simulink model "Wyparka3"  (R2018a)
settings: Solver=ode45  StartTime=0.0  StopTime=1600  FixedStep=0.1  RelTol=1e-6  EnableMultiTasking=on
libraries: simulink x7
settings Model: Creator=Maciek  LastModifiedBy=klukomski
settings DataIOCC: SaveFormat=Array  SignalLoggingSaveFormat=ModelDataLogs
settings OptimizationCC: ExpressionDepthLimit=2147483647  LifeSpan=inf
settings DebuggingCC: UnderspecifiedInitializationDetection=Classic  MergeDetectMultiDrivingBlocksExec=none  SolverPrmCheckMsg=warning  FcnCallInpInsideContextMsg=warning  StateNameClashWarn=warning  SFUnexpectedBacktrackingDiag=warning  SFNoUnconditionalDefaultTransitionDiag=warning  SFExecutionAtInitializationDiag=none
settings HardwareCC: ProdBitPerPointer=32  ProdBitPerSizeT=32  ProdBitPerPtrDiffT=32  ProdLargestAtomicFloat=None  ProdIntDivRoundTo=Undefined  ProdEndianess=Unspecified  ProdWordSize=32  ProdHWDeviceType=32-bit Generic
settings ModelReferenceCC: PropagateSignalLabelsOutOfModel=off
settings CodeAppCC: StateflowObjectComments=on
settings GRTTargetCC: TargetLangStandard=C89/C90 (ANSI)  GeneratePreprocessorConditionals=Disable all  CombineOutputUpdateFcns=off  GRTInterface=on
settings ConfigComp: CovMetricSettings=dw  CovHtmlReporting=on  CovSaveCumulativeToWorkspaceVar=on  CovSaveSingleToWorkspaceVar=on  CovExternalEMLEnable=off

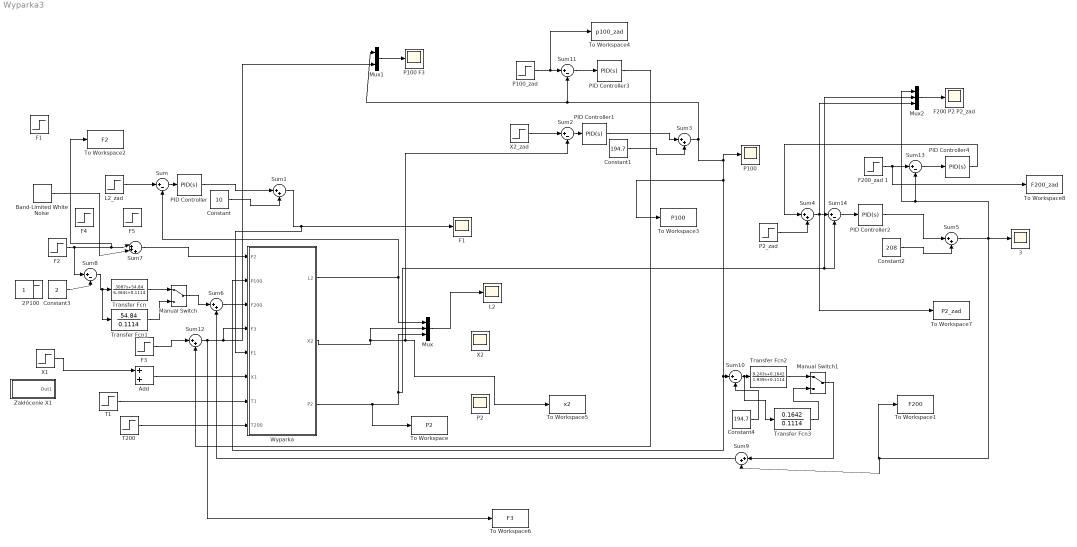
== system Wyparka3 ==
  "3 " : Scope
  Add : Sum
  Band-Limited White Noise : simulink/Sources/Band-Limited White Noise  Cov=[0.005]  Ts=2  seed=[23341]
  Constant : Constant  Value=10
  Constant1 : Constant  Value=194.7
  Constant2 : Constant  Value=208
  Constant3 : Constant  Value=2
  Constant4 : Constant  Value=194.7
  F1 : Step  Time=0  Before=10  After=9.9  SampleTime=0
  "F1 " : Scope
  F2 : Step  Time=200  Before=2  After=2  SampleTime=0
  F200 P2 P2_zad : Scope
  F200_zad 1 : Step  Time=700  Before=208  After=170  SampleTime=0
  F3 : Step  Time=0  Before=50  After=50  SampleTime=0
  F4 : Step  Time=300  After=-0.2  SampleTime=0
  F5 : Step  Time=2000  After=0.2  SampleTime=0
  L2 : Scope
  L2_zad : Step  Time=0  Before=1  SampleTime=0
  Manual Switch : ManualSwitch
  Manual Switch1 : ManualSwitch
  Mux : Mux  Inputs=3
  Mux1 : Mux  Inputs=2
  Mux2 : Mux  Inputs=3
  P100 : Step  Time=0  Before=194.7  After=194.7  SampleTime=0
  "P100 " : Scope
  P100 F3 : Scope
  "P100_zad " : Step  Time=100  Before=194.7  After=160  SampleTime=0
  P2 : Scope
  P2_zad : Step  Time=0  Before=50.5  After=50.5  SampleTime=0
  PID Controller : simulink/Continuous/PID Controller  Controller=PID  TimeDomain=Continuous-time  SampleTime=-1  IntegratorMethod=Forward Euler  FilterMethod=Forward Euler  Form=Parallel  UseFilter=on  ControllerParametersSource=internal  P=3.5228451242971  I=0.312459565800729  D=9.32811880876694  N=2.98089327538522  InitialConditionSource=internal  InitialConditionForIntegrator=0  InitialConditionForFilter=0  ExternalReset=none  LimitOutput=on  UpperSaturationLimit=10  LowerSaturationLimit=-10  LinearizeAsGain=on  AntiWindupMode=none  Kb=1  TrackingMode=off  Kt=1  PParamMin=[]  PParamMax=[]  IParamMin=[]  IParamMax=[]  DParamMin=[]  DParamMax=[]  NParamMin=[]  NParamMax=[]  KbParamMin=[]  KbParamMax=[]  KtParamMin=[]  KtParamMax=[]  POutMin=[]  POutMax=[]  IOutMin=[]  IOutMax=[]  DOutMin=[]  DOutMax=[]  NOutMin=[]  NOutMax=[]  KbOutMin=[]  KbOutMax=[]  KtOutMin=[]  KtOutMax=[]  IntegratorOutMin=[]  IntegratorOutMax=[]  FilterOutMin=[]  FilterOutMax=[]  SumOutMin=[]  SumOutMax=[]  SumI1OutMin=[]  SumI1OutMax=[]  SumI2OutMin=[]  SumI2OutMax=[]  SumI3OutMin=[]  SumI3OutMax=[]  SumDOutMin=[]  SumDOutMax=[]  SaturationOutMin=[]  SaturationOutMax=[]  IntegratorContinuousStateAttributes=''  IntegratorStateMustResolveToSignalObject=off  IntegratorRTWStateStorageClass=Auto  FilterContinuousStateAttributes=''  FilterStateMustResolveToSignalObject=off  FilterRTWStateStorageClass=Auto  DifferentiatorICPrevScaledInput=0  DifferentiatorOutMin=[]  DifferentiatorOutMax=[]  FilterDiffOutCoefMin=[]  FilterDiffOutCoefMax=[]  SumDenOutMin=[]  SumDenOutMax=[]  SumNumOutMin=[]  SumNumOutMax=[]  ReciprocalOutMin=[]  ReciprocalOutMax=[]  DivideOutMin=[]  DivideOutMax=[]  TunerSelectOption=Transfer Function Based (PID Tuner App)
  PID Controller1 : simulink/Continuous/PID Controller  Controller=PID  TimeDomain=Continuous-time  SampleTime=-1  IntegratorMethod=Forward Euler  FilterMethod=Forward Euler  Form=Parallel  UseFilter=on  ControllerParametersSource=internal  P=362.743618010896  I=63.281674643677  D=154.013703134731  N=5.51481835403711  InitialConditionSource=internal  InitialConditionForIntegrator=0  InitialConditionForFilter=0  ExternalReset=none  LimitOutput=on  UpperSaturationLimit=400-194.7  LowerSaturationLimit=-194.7  LinearizeAsGain=on  AntiWindupMode=none  Kb=1  TrackingMode=off  Kt=1  PParamMin=[]  PParamMax=[]  IParamMin=[]  IParamMax=[]  DParamMin=[]  DParamMax=[]  NParamMin=[]  NParamMax=[]  KbParamMin=[]  KbParamMax=[]  KtParamMin=[]  KtParamMax=[]  POutMin=[]  POutMax=[]  IOutMin=[]  IOutMax=[]  DOutMin=[]  DOutMax=[]  NOutMin=[]  NOutMax=[]  KbOutMin=[]  KbOutMax=[]  KtOutMin=[]  KtOutMax=[]  IntegratorOutMin=[]  IntegratorOutMax=[]  FilterOutMin=[]  FilterOutMax=[]  SumOutMin=[]  SumOutMax=[]  SumI1OutMin=[]  SumI1OutMax=[]  SumI2OutMin=[]  SumI2OutMax=[]  SumI3OutMin=[]  SumI3OutMax=[]  SumDOutMin=[]  SumDOutMax=[]  SaturationOutMin=[]  SaturationOutMax=[]  IntegratorContinuousStateAttributes=''  IntegratorStateMustResolveToSignalObject=off  IntegratorRTWStateStorageClass=Auto  FilterContinuousStateAttributes=''  FilterStateMustResolveToSignalObject=off  FilterRTWStateStorageClass=Auto  DifferentiatorICPrevScaledInput=0  DifferentiatorOutMin=[]  DifferentiatorOutMax=[]  FilterDiffOutCoefMin=[]  FilterDiffOutCoefMax=[]  SumDenOutMin=[]  SumDenOutMax=[]  SumNumOutMin=[]  SumNumOutMax=[]  ReciprocalOutMin=[]  ReciprocalOutMax=[]  DivideOutMin=[]  DivideOutMax=[]  TunerSelectOption=Transfer Function Based (PID Tuner App)
  PID Controller2 : simulink/Continuous/PID Controller  Controller=PID  TimeDomain=Continuous-time  SampleTime=-1  IntegratorMethod=Forward Euler  FilterMethod=Forward Euler  Form=Parallel  UseFilter=on  ControllerParametersSource=internal  P=-149.630552232494  I=-11.2071679575785  D=-131.417813851243  N=0.631872237421497  InitialConditionSource=internal  InitialConditionForIntegrator=0  InitialConditionForFilter=0  ExternalReset=none  LimitOutput=on  UpperSaturationLimit=400-208  LowerSaturationLimit=-208  LinearizeAsGain=on  AntiWindupMode=none  Kb=1  TrackingMode=off  Kt=1  PParamMin=[]  PParamMax=[]  IParamMin=[]  IParamMax=[]  DParamMin=[]  DParamMax=[]  NParamMin=[]  NParamMax=[]  KbParamMin=[]  KbParamMax=[]  KtParamMin=[]  KtParamMax=[]  POutMin=[]  POutMax=[]  IOutMin=[]  IOutMax=[]  DOutMin=[]  DOutMax=[]  NOutMin=[]  NOutMax=[]  KbOutMin=[]  KbOutMax=[]  KtOutMin=[]  KtOutMax=[]  IntegratorOutMin=[]  IntegratorOutMax=[]  FilterOutMin=[]  FilterOutMax=[]  SumOutMin=[]  SumOutMax=[]  SumI1OutMin=[]  SumI1OutMax=[]  SumI2OutMin=[]  SumI2OutMax=[]  SumI3OutMin=[]  SumI3OutMax=[]  SumDOutMin=[]  SumDOutMax=[]  SaturationOutMin=[]  SaturationOutMax=[]  IntegratorContinuousStateAttributes=''  IntegratorStateMustResolveToSignalObject=off  IntegratorRTWStateStorageClass=Auto  FilterContinuousStateAttributes=''  FilterStateMustResolveToSignalObject=off  FilterRTWStateStorageClass=Auto  DifferentiatorICPrevScaledInput=0  DifferentiatorOutMin=[]  DifferentiatorOutMax=[]  FilterDiffOutCoefMin=[]  FilterDiffOutCoefMax=[]  SumDenOutMin=[]  SumDenOutMax=[]  SumNumOutMin=[]  SumNumOutMax=[]  ReciprocalOutMin=[]  ReciprocalOutMax=[]  DivideOutMin=[]  DivideOutMax=[]  TunerSelectOption=Transfer Function Based (PID Tuner App)
  PID Controller3 : simulink/Continuous/PID Controller  Controller=PID  TimeDomain=Continuous-time  SampleTime=-1  IntegratorMethod=Forward Euler  FilterMethod=Forward Euler  Form=Parallel  UseFilter=on  ControllerParametersSource=internal  P=0  I=-0.02  D=0  N=100  InitialConditionSource=internal  InitialConditionForIntegrator=0  InitialConditionForFilter=0  ExternalReset=none  LimitOutput=on  UpperSaturationLimit=50  LowerSaturationLimit=-50  LinearizeAsGain=on  AntiWindupMode=none  Kb=1  TrackingMode=off  Kt=1  PParamMin=[]  PParamMax=[]  IParamMin=[]  IParamMax=[]  DParamMin=[]  DParamMax=[]  NParamMin=[]  NParamMax=[]  KbParamMin=[]  KbParamMax=[]  KtParamMin=[]  KtParamMax=[]  POutMin=[]  POutMax=[]  IOutMin=[]  IOutMax=[]  DOutMin=[]  DOutMax=[]  NOutMin=[]  NOutMax=[]  KbOutMin=[]  KbOutMax=[]  KtOutMin=[]  KtOutMax=[]  IntegratorOutMin=[]  IntegratorOutMax=[]  FilterOutMin=[]  FilterOutMax=[]  SumOutMin=[]  SumOutMax=[]  SumI1OutMin=[]  SumI1OutMax=[]  SumI2OutMin=[]  SumI2OutMax=[]  SumI3OutMin=[]  SumI3OutMax=[]  SumDOutMin=[]  SumDOutMax=[]  SaturationOutMin=[]  SaturationOutMax=[]  IntegratorContinuousStateAttributes=''  IntegratorStateMustResolveToSignalObject=off  IntegratorRTWStateStorageClass=Auto  FilterContinuousStateAttributes=''  FilterStateMustResolveToSignalObject=off  FilterRTWStateStorageClass=Auto  DifferentiatorICPrevScaledInput=0  DifferentiatorOutMin=[]  DifferentiatorOutMax=[]  FilterDiffOutCoefMin=[]  FilterDiffOutCoefMax=[]  SumDenOutMin=[]  SumDenOutMax=[]  SumNumOutMin=[]  SumNumOutMax=[]  ReciprocalOutMin=[]  ReciprocalOutMax=[]  DivideOutMin=[]  DivideOutMax=[]  TunerSelectOption=Transfer Function Based (PID Tuner App)
  PID Controller4 : simulink/Continuous/PID Controller  Controller=PID  TimeDomain=Continuous-time  SampleTime=-1  IntegratorMethod=Forward Euler  FilterMethod=Forward Euler  Form=Parallel  UseFilter=on  ControllerParametersSource=internal  P=0  I=-0.005  D=0  N=100  InitialConditionSource=internal  InitialConditionForIntegrator=0  InitialConditionForFilter=0  ExternalReset=none  LimitOutput=on  UpperSaturationLimit=49.5  LowerSaturationLimit=-50.5  LinearizeAsGain=on  AntiWindupMode=none  Kb=1  TrackingMode=off  Kt=1  PParamMin=[]  PParamMax=[]  IParamMin=[]  IParamMax=[]  DParamMin=[]  DParamMax=[]  NParamMin=[]  NParamMax=[]  KbParamMin=[]  KbParamMax=[]  KtParamMin=[]  KtParamMax=[]  POutMin=[]  POutMax=[]  IOutMin=[]  IOutMax=[]  DOutMin=[]  DOutMax=[]  NOutMin=[]  NOutMax=[]  KbOutMin=[]  KbOutMax=[]  KtOutMin=[]  KtOutMax=[]  IntegratorOutMin=[]  IntegratorOutMax=[]  FilterOutMin=[]  FilterOutMax=[]  SumOutMin=[]  SumOutMax=[]  SumI1OutMin=[]  SumI1OutMax=[]  SumI2OutMin=[]  SumI2OutMax=[]  SumI3OutMin=[]  SumI3OutMax=[]  SumDOutMin=[]  SumDOutMax=[]  SaturationOutMin=[]  SaturationOutMax=[]  IntegratorContinuousStateAttributes=''  IntegratorStateMustResolveToSignalObject=off  IntegratorRTWStateStorageClass=Auto  FilterContinuousStateAttributes=''  FilterStateMustResolveToSignalObject=off  FilterRTWStateStorageClass=Auto  DifferentiatorICPrevScaledInput=0  DifferentiatorOutMin=[]  DifferentiatorOutMax=[]  FilterDiffOutCoefMin=[]  FilterDiffOutCoefMax=[]  SumDenOutMin=[]  SumDenOutMax=[]  SumNumOutMin=[]  SumNumOutMax=[]  ReciprocalOutMin=[]  ReciprocalOutMax=[]  DivideOutMin=[]  DivideOutMax=[]  TunerSelectOption=Transfer Function Based (PID Tuner App)
  Sum{,2,8,10..11,13..14} (7 alike) : Sum  Inputs=|+-
  Sum{1,3..6,9,12} (7 alike) : Sum  Inputs=|++
  Sum7 : Sum  Inputs=|+++
  T1 : Step  Time=0  Before=40  After=40  SampleTime=0
  T200 : Step  Time=0  Before=25  After=25  SampleTime=0
  To Workspace : ToWorkspace  VariableName=P2  SampleTime=-1
      settings: Save2DSignal=2-D array (concatenate along first dimension)
  To Workspace1 : ToWorkspace  VariableName=F200  SampleTime=-1
      settings: Save2DSignal=2-D array (concatenate along first dimension)
  To Workspace2 : ToWorkspace  VariableName=F2  SampleTime=-1
      settings: Save2DSignal=2-D array (concatenate along first dimension)
  To Workspace3 : ToWorkspace  VariableName=P100  SampleTime=-1
      settings: Save2DSignal=2-D array (concatenate along first dimension)
  To Workspace4 : ToWorkspace  VariableName=p100_zad  SampleTime=-1
      settings: Save2DSignal=2-D array (concatenate along first dimension)
  To Workspace5 : ToWorkspace  VariableName=x2  SampleTime=-1
      settings: Save2DSignal=2-D array (concatenate along first dimension)
  To Workspace6 : ToWorkspace  VariableName=F3  SampleTime=-1
      settings: Save2DSignal=2-D array (concatenate along first dimension)
  To Workspace7 : ToWorkspace  VariableName=P2_zad  SampleTime=-1
      settings: Save2DSignal=2-D array (concatenate along first dimension)
  To Workspace8 : ToWorkspace  VariableName=F200_zad  SampleTime=-1
      settings: Save2DSignal=2-D array (concatenate along first dimension)
  Transfer Fcn : TransferFcn  Numerator=[3087 54.84]  Denominator=[6.364 0.1114]
  Transfer Fcn1 : TransferFcn  Numerator=[54.84]  Denominator=[0.1114]
  Transfer Fcn2 : TransferFcn  Numerator=[9.243 0.1642]  Denominator=[1.939 0.1114]
  Transfer Fcn3 : TransferFcn  Numerator=[0.1642]  Denominator=[0.1114]
  Wyparka : Subsystem
  X1 : Step  Time=0  Before=5  After=5  SampleTime=0
  X2 : Scope
  X2_zad : Step  Time=0  Before=25  After=25  SampleTime=0
  Zakłócenie X1 : Subsystem
  2 : Constant  IOType=siggen
  wires:
  Wyparka/1(L2) -> Sum/2, Mux/1
  T1/1 -> Wyparka/7(T1)
  T200/1 -> Wyparka/8(T200)
  X1/1 -> Add/1
  Add/1 -> Wyparka/6(X1)
  L2_zad/1 -> Sum/1
  Sum/1 -> PID Controller/1
  PID Controller/1 -> Sum1/1
  Constant/1 -> Sum1/2
  Sum1/1 -> Wyparka/5(F1), "F1 "/1
  Wyparka/2(X2) -> To Workspace5/1, Sum2/2, Mux/2
  Wyparka/3(P2) -> To Workspace/1, Sum14/2, Mux2/2, Mux/3
  Mux/1 -> L2/1
  F2/1 -> Sum8/1, To Workspace2/1, Sum7/1
  X2_zad/1 -> Sum2/1
  Sum2/1 -> PID Controller1/1
  Constant1/1 -> Sum3/2
  P2_zad/1 -> Sum4/2
  Constant2/1 -> Sum5/2
  Sum6/1 -> Wyparka/3(F200)
  Transfer Fcn/1 -> Manual Switch/1
  Manual Switch/1 -> Sum6/1
  Sum7/1 -> Wyparka/1(F2)
  Sum8/1 -> Transfer Fcn1/1, Transfer Fcn/1
  Constant3/1 -> Sum8/2
  Sum3/1 -> Sum11/2, Mux1/1, To Workspace3/1, Sum10/1, Wyparka/2(P100), "P100 "/1
  Transfer Fcn2/1 -> Manual Switch1/1
  Sum9/1 -> Sum6/2
  Manual Switch1/1 -> Sum9/1
  PID Controller2/1 -> Sum5/1
  Sum10/1 -> Transfer Fcn3/1, Transfer Fcn2/1
  Constant4/1 -> Sum10/2
  Transfer Fcn3/1 -> Manual Switch1/2
  PID Controller1/1 -> Sum3/1
  Sum11/1 -> PID Controller3/1
  "P100_zad "/1 -> To Workspace4/1, Sum11/1
  PID Controller3/1 -> Sum12/2
  Sum12/1 -> To Workspace6/1, Mux1/2, Wyparka/4(F3)
  F3/1 -> Sum12/1
  Mux1/1 -> P100 F3/1
  Sum13/1 -> PID Controller4/1
  Sum5/1 -> "3 "/1, Mux2/1, Sum13/2, Sum9/2, To Workspace1/1
  F200_zad 1/1 -> To Workspace8/1, Sum13/1
  Mux2/1 -> F200 P2 P2_zad/1
  Sum14/1 -> PID Controller2/1
  Sum4/1 -> To Workspace7/1, Mux2/3, Sum14/1
  Transfer Fcn1/1 -> Manual Switch/2
  PID Controller4/1 -> Sum4/1
  Band-Limited White Noise/1 -> Sum7/2

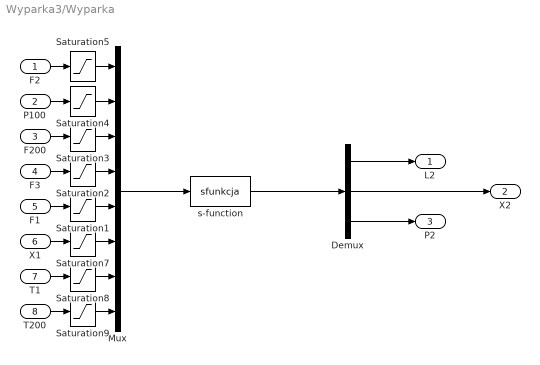
== system Wyparka3/Wyparka ==
  F2 : Inport
  P100 : Inport  Port=2
  F200 : Inport  Port=3
  F3 : Inport  Port=4
  F1 : Inport  Port=5
  X1 : Inport  Port=6
  T1 : Inport  Port=7
  T200 : Inport  Port=8
  Demux : Demux  Outputs=3
  Mux : Mux  Inputs=8
  Saturation1 : Saturate  UpperLimit=20  LowerLimit=0
  Saturation2 : Saturate  UpperLimit=100  LowerLimit=0
  Saturation3 : Saturate  UpperLimit=400  LowerLimit=0
  Saturation4 : Saturate  UpperLimit=400  LowerLimit=0
  Saturation5 : Saturate  UpperLimit=4  LowerLimit=0
  Saturation7 : Saturate  UpperLimit=100  LowerLimit=0
  Saturation8 : Saturate  UpperLimit=90  LowerLimit=5
  Saturation9 : Saturate  UpperLimit=90  LowerLimit=5
  s-function : S-Function  FunctionName=sfunkcja  SFunctionDeploymentMode=off  EnableBusSupport=off
  L2 : Outport
  X2 : Outport  Port=2
  P2 : Outport  Port=3
  wires:
  s-function/1 -> Demux/1
  Mux/1 -> s-function/1
  P100/1 -> Saturation4/1
  Demux/1 -> L2/1
  F200/1 -> Saturation3/1
  Demux/2 -> X2/1
  F3/1 -> Saturation2/1
  Demux/3 -> P2/1
  F1/1 -> Saturation1/1
  X1/1 -> Saturation7/1
  T1/1 -> Saturation8/1
  T200/1 -> Saturation9/1
  F2/1 -> Saturation5/1
  Saturation1/1 -> Mux/5
  Saturation2/1 -> Mux/4
  Saturation3/1 -> Mux/3
  Saturation4/1 -> Mux/2
  Saturation5/1 -> Mux/1
  Saturation7/1 -> Mux/6
  Saturation8/1 -> Mux/7
  Saturation9/1 -> Mux/8

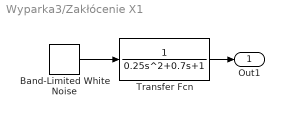
== system Wyparka3/Zakłócenie X1 ==
  Band-Limited White Noise : simulink/Sources/Band-Limited White Noise  Cov=[0.1]  Ts=0.05  seed=[23341]
  Transfer Fcn : TransferFcn  Denominator=[0.25 0.7 1]
  Out1 : Outport
  wires:
  Band-Limited White Noise/1 -> Transfer Fcn/1
  Transfer Fcn/1 -> Out1/1
